simulink model "clik_inverse"  (R2022b)
settings: Solver=ode1  StartTime=0.0  StopTime=4  FixedStep=0.001  RelTol=1e-3
undefined symbols (not defined in the file or in its folder): DiscIntNeverNeededParam, q0, Tc
settings Model: Creator=Xp  LastModifiedBy=shubham
settings SolverCC: AlgebraicLoopSolver=TrustRegion
settings DataIOCC: LimitDataPoints=on  SaveFormat=Array  SignalLoggingSaveFormat=ModelDataLogs  ReturnWorkspaceOutputs=off
settings OptimizationCC: ExpressionDepthLimit=2147483647  InitFltsAndDblsToZero=on  LifeSpan=inf
settings DebuggingCC: SaveWithParameterizedLinksMsg=none  UnderspecifiedInitializationDetection=Classic  MergeDetectMultiDrivingBlocksExec=none  SolverPrmCheckMsg=warning  MultiTaskDSMMsg=warning  MultiTaskCondExecSysMsg=none  FcnCallInpInsideContextMsg=warning  UnconnectedInputMsg=warning  UnconnectedOutputMsg=warning  UnconnectedLineMsg=warning  StateNameClashWarn=warning  SFUnexpectedBacktrackingDiag=warning  SFNoUnconditionalDefaultTransitionDiag=warning  SFExecutionAtInitializationDiag=none  SFMachineParentedDataDiag=warning  ArithmeticOperatorsInVariantConditions=warning
settings HardwareCC: ProdBitPerPointer=32  ProdBitPerSizeT=32  ProdBitPerPtrDiffT=32  ProdLargestAtomicFloat=None  ProdIntDivRoundTo=Undefined  ProdEndianess=Unspecified  ProdWordSize=32  ProdHWDeviceType=32-bit Generic
settings ModelReferenceCC: EnableRefExpFcnMdlSchedulingChecks=on  PropagateSignalLabelsOutOfModel=off
settings SFSimCC: CustomCodeUndefinedFunction=UseInterfaceOnly
settings RTWCC: DLArmComputeVersion=19.05
settings CodeAppCC: StateflowObjectComments=on
settings GRTTargetCC: TargetLangStandard=C89/C90 (ANSI)  CombineOutputUpdateFcns=off  GRTInterface=on
settings ConfigComp: CovMetricSettings=dw  CovSaveCumulativeToWorkspaceVar=on  CovSaveSingleToWorkspaceVar=on

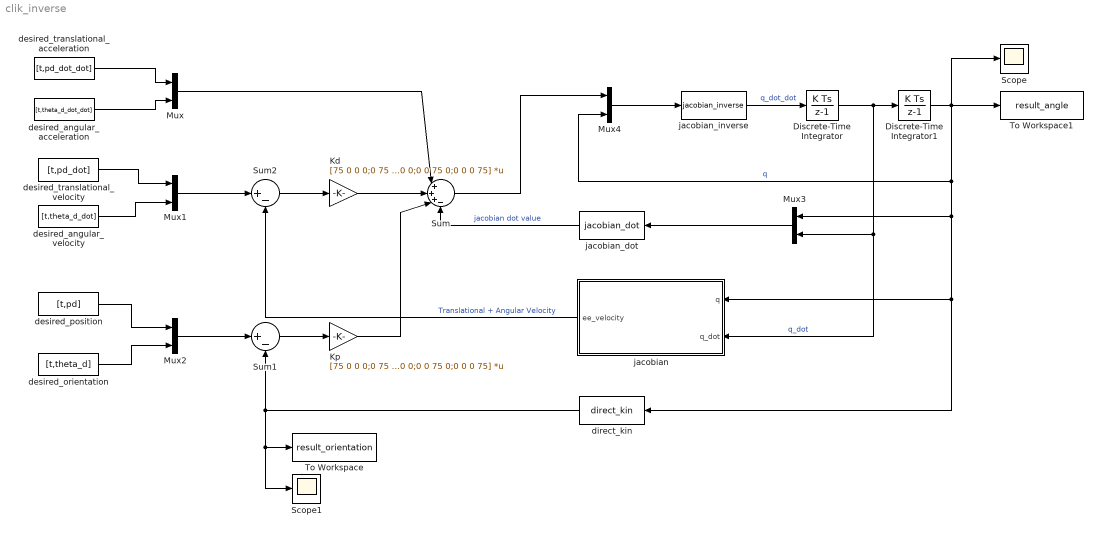
== system clik_inverse ==
  Discrete-Time Integrator : DiscreteIntegrator  InitialCondition=[0;0;0;0]  SampleTime=Tc  ICPrevOutput=DiscIntNeverNeededParam  ICPrevScaledInput=DiscIntNeverNeededParam
  Discrete-Time Integrator1 : DiscreteIntegrator  InitialCondition=q0  SampleTime=Tc  LimitOutput=on  UpperSaturationLimit=[inf, inf, 1, inf]  LowerSaturationLimit=[-inf, -inf, -0.25, -inf]  ICPrevOutput=DiscIntNeverNeededParam  ICPrevScaledInput=DiscIntNeverNeededParam
  Kd : Gain  Gain=[75 0 0 0;0 75 0 0;0 0 75 0;0 0 0 75]  Multiplication=Matrix(K*u)
  Kp : Gain  Gain=[75 0 0 0;0 75 0 0;0 0 75 0;0 0 0 75]  Multiplication=Matrix(K*u)
  Mux{,1..4} (5 alike) : Mux  Inputs=2
  Scope : Scope
  Scope1 : Scope
  Sum : Sum  Inputs=|+++-
  Sum1 : Sum  Inputs=|+-
  Sum2 : Sum  Inputs=|+-
  To Workspace : ToWorkspace  VariableName=result_orientation  SampleTime=-1
  To Workspace1 : ToWorkspace  VariableName=result_angle  SampleTime=-1
      settings: Save2DSignal=2-D array (concatenate along first dimension)
  desired_angular_acceleration : FromWorkspace  VariableName=[t,theta_d_dot_dot]
  desired_angular_velocity : FromWorkspace  VariableName=[t,theta_d_dot]
  desired_orientation : FromWorkspace  VariableName=[t,theta_d]
  desired_position : FromWorkspace  VariableName=[t,pd]
  "desired_translational_acceleration " : FromWorkspace  VariableName=[t,pd_dot_dot]
  desired_translational_velocity : FromWorkspace  VariableName=[t,pd_dot]
  direct_kin : MATLABFcn  MATLABFcn=direct_kin  OutputDimensions=4
  "jacobian " : MATLAB Function  TreatAsAtomicUnit=on
  jacobian_dot : MATLABFcn  MATLABFcn=jacobian_dot  OutputDimensions=4
  jacobian_inverse : MATLABFcn  MATLABFcn=jacobian_inverse  OutputDimensions=4
  wires:
  jacobian_dot/1 -> Sum/4  "jacobian dot value"
  desired_orientation/1 -> Mux2/2
  Mux2/1 -> Sum1/1
  Discrete-Time Integrator/1 -> Discrete-Time Integrator1/1, "jacobian "/2(q_dot), Mux3/2  "q_dot"
  Kd/1 -> Sum/2
  direct_kin/1 -> Scope1/1, To Workspace/1, Sum1/2
  Mux3/1 -> jacobian_dot/1
  desired_translational_velocity/1 -> Mux1/1
  desired_position/1 -> Mux2/1
  Discrete-Time Integrator1/1 -> To Workspace1/1, Scope/1, Mux4/2, Mux3/1, "jacobian "/1(q), direct_kin/1  "q"
  desired_angular_velocity/1 -> Mux1/2
  Mux1/1 -> Sum2/1
  Kp/1 -> Sum/3
  Sum2/1 -> Kd/1
  Mux4/1 -> jacobian_inverse/1
  jacobian_inverse/1 -> Discrete-Time Integrator/1  "q_dot_dot"
  "jacobian "/1(ee_velocity) -> Sum2/2  "Translational + Angular Velocity"
  Sum1/1 -> Kp/1
  Mux/1 -> Sum/1
  "desired_translational_acceleration "/1 -> Mux/1
  desired_angular_acceleration/1 -> Mux/2
  Sum/1 -> Mux4/1

== matlab function clik_inverse/jacobian  ==
  data: q input; ee_velocity output; q_dot input
function ee_velocity= fcn(q,q_dot)
    %input parameters
    theta1=q(1);
    theta2=q(2);
    
    %robot parameters
    a1=0.5;
    a2=0.5;
    
    Jacobian=[-a2*sin(theta1 + theta2) - a1*sin(theta1), -a2*sin(theta1 + theta2), 0, 0; 
        a2*cos(theta1 + theta2) + a1*cos(theta1), a2*cos(theta1 + theta2), 0,0; 
        0, 0, -1, 0;
        1, 1, 0, 1];
    
    ee_velocity=Jacobian*q_dot;

end
